simulink model "servodistlib"  (R2016a)
settings: Solver=VariableStepAuto  StartTime=0.0  StopTime=10.0  RelTol=1e-3
libraries: simulink x3
settings Model: Creator=jordan  LastModifiedBy=jordan

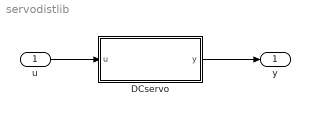
== system servodistlib ==
  u : Inport
  DCservo : Subsystem
  y : Outport
  wires:
  u/1 -> DCservo/1(u)
  DCservo/1(y) -> y/1

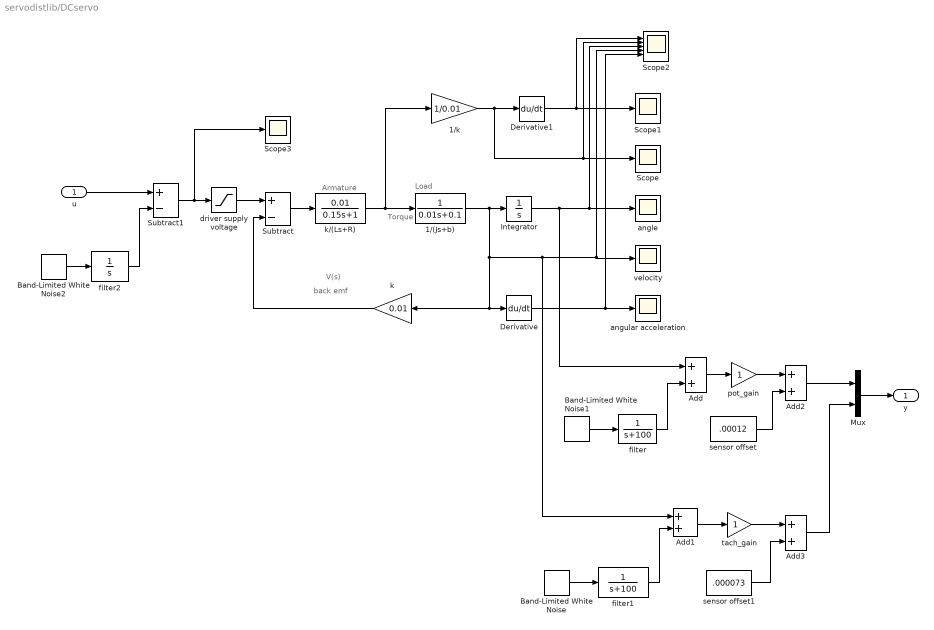
== system servodistlib/DCservo ==
  note: back emf
  note: Armature
  note: Torque
  note: Load
  note: V(s)
  u : Inport
  1/(Js+b) : TransferFcn  Denominator=[0.01 0.1]
  1/k : Gain  Gain=1/0.01
  Add{,1..3} (4 alike) : Sum
  Band-Limited White Noise : simulink/Sources/Band-Limited White Noise  Cov=[0.000002]  Ts=0.1  seed=[24341]
  Band-Limited White Noise1 : simulink/Sources/Band-Limited White Noise  Cov=[0.000002]  Ts=0.1  seed=[23341]
  Band-Limited White Noise2 : simulink/Sources/Band-Limited White Noise  Cov=[0.0002]  Ts=0.1  seed=[23341]
  Derivative : Derivative
  Derivative1 : Derivative
  Integrator : Integrator
  Mux : Mux  Inputs=2
  Scope : Scope
  Scope1 : Scope
  Scope2 : Scope  NumInputPorts=5
  Scope3 : Scope
  Subtract : Sum  Inputs=+-
  Subtract1 : Sum  Inputs=+-
  angle : Scope
  angular acceleration : Scope
  driver supply voltage : Saturate  UpperLimit=12  LowerLimit=-12
  filter : TransferFcn  Denominator=[1 100]
  filter1 : TransferFcn  Denominator=[1 100]
  filter2 : TransferFcn  Denominator=[1 0]
  k : Gain  Gain=0.01
  k/(Ls+R) : TransferFcn  Numerator=[0.01]  Denominator=[0.15 1]
  pot_gain : Gain
  sensor offset : Constant  Value=.00012
  sensor offset1 : Constant  Value=.000073
  tach_gain : Gain
  velocity : Scope
  y : Outport
  wires:
  k/(Ls+R)/1 -> 1/(Js+b)/1, 1/k/1
  1/(Js+b)/1 -> Integrator/1, velocity/1, Scope2/4, Add1/1, Derivative/1, k/1
  Integrator/1 -> angle/1, Scope2/3, Add/1
  k/1 -> Subtract/2
  Subtract/1 -> k/(Ls+R)/1
  Derivative/1 -> angular acceleration/1, Scope2/5
  1/k/1 -> Scope2/2, Scope/1, Derivative1/1
  Derivative1/1 -> Scope1/1, Scope2/1
  Mux/1 -> y/1
  driver supply voltage/1 -> Subtract/1
  Add/1 -> pot_gain/1
  Add1/1 -> tach_gain/1
  Band-Limited White Noise1/1 -> filter/1
  Band-Limited White Noise/1 -> filter1/1
  filter/1 -> Add/2
  filter1/1 -> Add1/2
  pot_gain/1 -> Add2/1
  Add2/1 -> Mux/1
  tach_gain/1 -> Add3/1
  Add3/1 -> Mux/2
  sensor offset/1 -> Add2/2
  sensor offset1/1 -> Add3/2
  u/1 -> Subtract1/1
  Subtract1/1 -> Scope3/1, driver supply voltage/1
  Band-Limited White Noise2/1 -> filter2/1
  filter2/1 -> Subtract1/2
